simulink model "verify_Storage_Type_3_CONF_mdl"  (R2016b)
settings: Solver=ode45  StartTime=0  StopTime=24*3600  MaxStep=600  RelTol=1e-3  EnableMultiTasking=on
undefined symbols (not defined in the file or in its folder): path_carnot
libraries: carnot x8
settings Model: Creator=drhf  LastModifiedBy=drhf
settings DataIOCC: SaveFormat=Array  SignalLoggingSaveFormat=ModelDataLogs
settings OptimizationCC: ExpressionDepthLimit=2147483647  LifeSpan=inf
settings DebuggingCC: UnderspecifiedInitializationDetection=Classic  MergeDetectMultiDrivingBlocksExec=none  SolverPrmCheckMsg=warning  FcnCallInpInsideContextMsg=warning  StateNameClashWarn=warning  SFUnexpectedBacktrackingDiag=warning  SFNoUnconditionalDefaultTransitionDiag=warning  SFExecutionAtInitializationDiag=none
settings HardwareCC: ProdBitPerPointer=32  ProdBitPerSizeT=32  ProdBitPerPtrDiffT=32  ProdLargestAtomicFloat=None  ProdIntDivRoundTo=Undefined  ProdEndianess=Unspecified  ProdWordSize=32  ProdHWDeviceType=32-bit Generic
settings ModelReferenceCC: PropagateSignalLabelsOutOfModel=off
settings GRTTargetCC: TargetLangStandard=C89/C90 (ANSI)  GeneratePreprocessorConditionals=Disable all  CombineOutputUpdateFcns=off  GRTInterface=on
settings ConfigComp: CovMetricSettings=dw  CovHtmlReporting=on  CovSaveCumulativeToWorkspaceVar=on  CovSaveSingleToWorkspaceVar=on  CovExternalEMLEnable=off

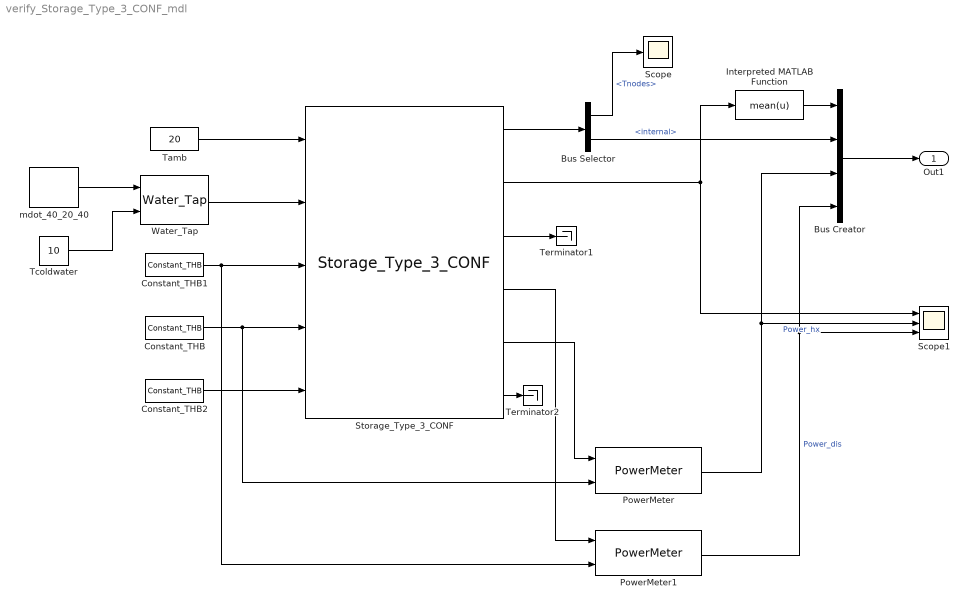
== system verify_Storage_Type_3_CONF_mdl ==
  Bus Creator : BusCreator  Inputs=4
  Bus Selector : BusSelector  OutputSignals=Tnodes,energy.internal
  Constant_THB : carnot/Source/Simple/Constant_THB  t=50  mdot=200/3600  p=1e5  mID=No Pressure Drop  fluid=Water (Constant 20°C)  mix=0  mix2=0  mix3=0  dia=0.02  hgt=0
  Constant_THB1 : carnot/Source/Simple/Constant_THB  t=60  mdot=600/3600  p=1e5  mID=No Pressure Drop  fluid=Water (Constant 20°C)  mix=0  mix2=0  mix3=0  dia=0.02  hgt=0
  Constant_THB2 : carnot/Source/Simple/Constant_THB  t=50  mdot=0  p=1e5  mID=No Pressure Drop  fluid=Water (Constant 20°C)  mix=0  mix2=0  mix3=0  dia=0.02  hgt=0
  Interpreted MATLAB Function : MATLABFcn  MATLABFcn=mean(u)
  PowerMeter : carnot/Control/PowerMeter
  PowerMeter1 : carnot/Control/PowerMeter
  Scope : Scope
  Scope1 : Scope  NumInputPorts=3
  Storage_Type_3_CONF : carnot/Storage/Thermal/Storage_Type_3_CONF  t0=[10:5:55]  hgt=1.6836  stgtype=3  tini=[10 15 20 25 30 35 40 45 50 55]  mpts=[1 2 3 4 5 6 7 8 9 10]  PathName=fullfile(path_carnot('libsl'),'Storage','Thermal','Storage_Type_3_CONF','parameter_set')  FileName='StorageType3_400_L.mat'  userPath=off  userParam=off  uwall=1  ubot=1  utop=1  axcond=1  volume=0.4  dia=0.55  standing=standing cylinder  nodes=10  mpoints=10  Tsensor=[0.1 0.5 0.7]  hx1inlet=0.8  hx1outlet=0.6  hx1dia=0.03  hx1uac=50  hx1uam=0.15  hx1uat=0.6  hx1dpqua=20  hx1dplin=20  hx2inlet=0.4  hx2outlet=0  hx2dia=0.03  hx2uac=100  hx2uam=0.15  hx2uat=0.6  hx2dplin=30  hx2dpqua=30  pipe1inlet=0.02  pipe1outlet=0.98  pipe1dia=0.03  pipe2inlet=0.6  pipe2outlet=1  pipe2dia=0.03
  Tamb : Constant  Value=20
  Tcoldwater : Constant  Value=10
  Terminator1 : Terminator
  Terminator2 : Terminator
  Water_Tap : carnot/Load/Hot_Water_Tapping/Water_Tap  dia=0.02  p=2e5
  mdot_40_20_40 : carnot/Load/Hot_Water_Tapping/mdot_40_20_40  period=24*3600  rep_seq_t=[7 12 19]*3600  rep_seq_d=[0.2 0.1 0.2]*3600  rep_seq_y=[1 1 1]*200/1800
  Out1 : Outport
  wires:
  Bus Creator/1 -> Out1/1
  Tamb/1 -> Storage_Type_3_CONF/1
  Constant_THB1/1 -> PowerMeter1/2, Storage_Type_3_CONF/3
  Constant_THB/1 -> PowerMeter/2, Storage_Type_3_CONF/4
  Storage_Type_3_CONF/1 -> Bus Selector/1
  Storage_Type_3_CONF/5 -> PowerMeter/1
  Storage_Type_3_CONF/4 -> PowerMeter1/1
  PowerMeter/1 -> Bus Creator/3, Scope1/2  "Power_hx"
  PowerMeter1/1 -> Bus Creator/4, Scope1/3  "Power_dis"
  Storage_Type_3_CONF/2 -> Interpreted MATLAB Function/1, Scope1/1
  mdot_40_20_40/1 -> Water_Tap/1
  Tcoldwater/1 -> Water_Tap/2
  Water_Tap/1 -> Storage_Type_3_CONF/2
  Storage_Type_3_CONF/3 -> Terminator1/1
  Bus Selector/2 -> Bus Creator/2  "<internal>"
  Constant_THB2/1 -> Storage_Type_3_CONF/5
  Storage_Type_3_CONF/6 -> Terminator2/1
  Interpreted MATLAB Function/1 -> Bus Creator/1
  Bus Selector/1 -> Scope/1  "<Tnodes>"
